simulink model "part2_MAIN_2019_for_ayon_because_he_cant_update_his_matlab"  (R2019a)
settings: Solver=FixedStepAuto  StartTime=0.0  StopTime=300  FixedStep=0.1  RelTol=1e-3
values from neighbouring files (symbols this model uses):
  Af = diag(ti)    [init.m]    (also in init_old.m)
  Aw = [zeros(3) eye(3) ... (first row only)    [get_observer_parameters.m]
  B = [thr1 thr2_x thr2_y thr3 thr4_x thr4_y thr5_x thr5_y]    [B_redistributed.m]    (also in check_alg.m = [1 2 3 4 5 6 7 8; get_observer_parameters.m = [zeros(6,3);zeros(3,3);zeros(3,3);inv(M)])
  change_position_time = 1200    [init.m]    (also in init_old.m)
  Cw = [zeros(3) eye(3)]    [get_observer_parameters.m]
  D = Damping    [init.m]    (also in init_old.m)
  Damping = diag([2.6486e5, 8.8164e5, 3.3774e8])    [init.m]    (also in init_old.m)
  direction_limit = pi/36    (= 0.0872664625997)    [init.m]    (also in init_old.m)
  direction_time_constant = 100    [init.m]    (also in init_old.m)
  dt = 0.1    [get_observer_parameters.m]
  E = [Ew, zeros(6,3) ... (first row only)    [get_observer_parameters.m]
  Gamma = diag(omega_is)    [init.m]    (also in init_old.m)
  gust_limit = 40    [init.m]    (also in init_old.m)
  H = [Cw, eye(3), zeros(3,3) zeros(3,3)]    [get_observer_parameters.m]    (also in quadprog.m = 2*diag([w.' w.' q.' q.' w_alpha.' w_alpha.']); quadprog_basic.m = 2*diag([w.' w.' q.' q.']); quadprog_false.m = 2*diag([w.' w.' q.' q.' w_alpha.' w_alpha.']))
  height = 3    [init.m]    (also in init_old.m)
  inv_M = inv(M)    [get_observer_parameters.m]
  inv_Tb = inv(Tb)    [get_observer_parameters.m]
  kappa = 0.003    [init.m]    (also in init_old.m)
  kappa2 = 0.0026    [init.m]    (also in init_old.m)
  Kd = [1660451.40544401; 3920391.80535684; 1605063439.04156]    [init.m]    (also in init_old.m)
  Ki = [137.081306245593; 3163.274947400198; 335358.448218978]    [init.m]    (also in init_old.m)
  Kp = [75459.3345349083; 277551.73586971; 120744473.878042]    [init.m]    (also in init_old.m)
  L = 1800    [init.m]    (also in init_old.m)
  M = Mass    [init.m]    (also in init_old.m)
  mean_wind_direction = pi    (= 3.14159265359)    [init.m]    (also in init_old.m)
  observer_type = 0    [init.m]    (also in init_old.m)
  Omega = diag([omega_n, omega_n, omega_n])    [get_observer_parameters.m]    (also in init.m = diag(2*omega_is.*zeta_is); init_old.m = diag(2*omega_is.*zeta_is))
  Q = diag([0.1,0.1,pi/180,1e6,1e6,1e9])*10e3    [get_observer_parameters.m]
  R = diag([1,0.1,0.1*pi/180])*10e-3    [get_observer_parameters.m]
  simulation = 7    [init.m]    (also in init_old.m = 1)
  slow_varying_limit = 1    [init.m]    (also in init_old.m)
  slow_varying_time_constant = 100    [init.m]    (also in init_old.m)
  TAU = dt*E    [get_observer_parameters.m]
  Tb = 0.1 * eye(3)    [get_observer_parameters.m]
  thruster_type = 0    [init.m]    (also in init_old.m)
  u10 = 12    [init.m]    (also in init_old.m)
  vessel =     [test.mat]
  wind = 1    [init.m]    (also in init_old.m)
undefined symbols (not defined in the file or in its folder): Hoerner, ModelParams, npf, Param, thrusters, WaveModel
libraries: simulink x49, dspsigops x39, marine_hydro x14, marine_gnc x7
(part 6 of 9)

== system part2_MAIN_2019_for_ayon_because_he_cant_update_his_matlab/Simulation 5/Observer/Passive Non-Linear ==
  note: eta_observer
  note: nu_observer
  note: Bias Estimator
  note: Wave Estimator: 1st order wave-induced motion
  y : Inport
  tau_est : Inport  Port=2
  Add : Sum
  Add1 : Sum  Inputs=++-
  Aw : Gain  Gain=WaveModel.A_w  Multiplication=Matrix(K*u)
  Cw : Gain  Gain=WaveModel.C_w  Multiplication=Matrix(K*u)
  Damping : Gain  Gain=Damping  Multiplication=Matrix(K*u)
  Integrator{,1..3} (4 alike) : Integrator
  K1 : Gain  Gain=npf.K_1  Multiplication=Matrix(K*u)
  K2 : Gain  Gain=npf.K_2  Multiplication=Matrix(K*u)
  K3 : Gain  Gain=npf.K_3  Multiplication=Matrix(K*u)
  K4 : Gain  Gain=npf.K_4  Multiplication=Matrix(K*u)
  M_inv : Gain  Gain=inv(ModelParams.Mass)  Multiplication=Matrix(K*u)
  Matrix Multiply : Product  Multiplication=Matrix(*)
  Matrix Multiply1 : Product  Multiplication=Matrix(*)
  Matrix Multiply2 : Product  Multiplication=Matrix(*)
  R_psi : MATLAB Function  TreatAsAtomicUnit=on
  R_psi_T : MATLAB Function  TreatAsAtomicUnit=on
  Subsystem : Subsystem
  Sum : Sum  Inputs=|++
  Sum1 : Sum  Inputs=|+-
  Sum2 : Sum  Inputs=|++
  Sum3 : Sum  Inputs=|++
  Sum4 : Sum  Inputs=|+-
  inv(Tb) : Gain  Gain=inv(Param.Tb)  Multiplication=Matrix(K*u)
  eta_hat : Outport
  nu_hat : Outport  Port=2
  wires:
  Matrix Multiply/1 -> Sum/1
  Matrix Multiply1/1 -> Add/2
  Matrix Multiply2/1 -> Add1/1  "R'b_hat"
  R_psi_T/1(y) -> Matrix Multiply/1, Matrix Multiply2/2
  Add1/1 -> M_inv/1
  Damping/1 -> Add1/3
  R_psi/1(y) -> Matrix Multiply1/1
  Sum/1 -> Add1/2  "R'k4y + tau"
  Add/1 -> Integrator3/1  "eta_hat_dot"
  inv(Tb)/1 -> Sum1/2
  y/1 -> Subsystem/1(y), Sum4/1  "y"
  Aw/1 -> Sum2/2
  K3/1 -> Sum1/1
  Cw/1 -> Sum3/1
  Integrator1/1 -> Cw/1, Aw/1  "zeta_hat"
  Sum1/1 -> Integrator2/1  "b_hat_dot"
  Integrator/1 -> nu_hat/1, Damping/1, Matrix Multiply1/2  "nu_hat"
  Sum4/1 -> K1/1, K2/1, K3/1, K4/1  "y_obs"
  Sum3/1 -> Sum4/2  "y_hat"
  Integrator3/1 -> eta_hat/1, Sum3/2  "eta_hat"
  Sum2/1 -> Integrator1/1
  K2/1 -> Add/1
  K4/1 -> Matrix Multiply/2
  M_inv/1 -> Integrator/1  "nu_hat_dot"
  Integrator2/1 -> inv(Tb)/1, Matrix Multiply2/1  "b_hat"
  tau_est/1 -> Sum/2
  K1/1 -> Sum2/1
  Subsystem/1(Out1) -> R_psi/1(u), R_psi_T/1(u)

== system part2_MAIN_2019_for_ayon_because_he_cant_update_his_matlab/Simulation 5/Observer/Subsystem ==
  In1 : Inport
  Demux : Demux  Outputs=6
  Mux : Mux  Inputs=3
  Terminator : Terminator
  Terminator1 : Terminator
  Terminator2 : Terminator
  Out1 : Outport
  wires:
  Mux/1 -> Out1/1
  Demux/6 -> Mux/3
  Demux/5 -> Terminator2/1
  Demux/2 -> Mux/2
  Demux/1 -> Mux/1
  Demux/3 -> Terminator/1
  In1/1 -> Demux/1
  Demux/4 -> Terminator1/1

== system part2_MAIN_2019_for_ayon_because_he_cant_update_his_matlab/Simulation 5/Reference Model/Simulation Selector ==
  Simulation 4 : Subsystem
  Out1 : Outport
  wires:
  Simulation 4/1(Out1) -> Out1/1

== system part2_MAIN_2019_for_ayon_because_he_cant_update_his_matlab/Simulation 5/Thrust Allocation/Unwrap ==
  alpha : Inport
  Demux : Demux  Outputs=5
  Mux : Mux  Inputs=5
  Unwrap : dspsigops/Unwrap  tol=pi  InputProcessing=Columns as channels (frame based)  running=off
  Unwrap1 : dspsigops/Unwrap  tol=pi  InputProcessing=Columns as channels (frame based)  running=off
  Unwrap2 : dspsigops/Unwrap  tol=pi  InputProcessing=Columns as channels (frame based)  running=off
  alpha [rad] : Outport
  wires:
  alpha/1 -> Demux/1
  Mux/1 -> alpha [rad]/1
  Demux/1 -> Mux/1
  Demux/4 -> Unwrap2/1
  Unwrap2/1 -> Mux/4
  Demux/5 -> Unwrap/1
  Unwrap/1 -> Mux/5
  Demux/3 -> Mux/3
  Demux/2 -> Unwrap1/1
  Unwrap1/1 -> Mux/2

== system part2_MAIN_2019_for_ayon_because_he_cant_update_his_matlab/Simulation 5/Thrust Allocation/Unwrap1 ==
  alpha : Inport
  Demux : Demux  Outputs=5
  Mux : Mux  Inputs=5
  Unwrap : dspsigops/Unwrap  tol=pi  InputProcessing=Columns as channels (frame based)  running=off
  Unwrap1 : dspsigops/Unwrap  tol=pi  InputProcessing=Columns as channels (frame based)  running=off
  Unwrap2 : dspsigops/Unwrap  tol=pi  InputProcessing=Columns as channels (frame based)  running=off
  alpha [rad] : Outport
  wires:
  Unwrap1/1 -> Mux/2
  Demux/2 -> Unwrap1/1
  Demux/3 -> Mux/3
  Unwrap/1 -> Mux/5
  Demux/5 -> Unwrap/1
  Unwrap2/1 -> Mux/4
  Demux/4 -> Unwrap2/1
  Demux/1 -> Mux/1
  Mux/1 -> alpha [rad]/1
  alpha/1 -> Demux/1

== system part2_MAIN_2019_for_ayon_because_he_cant_update_his_matlab/Simulation 5/Wind/V_w1 ==
  " " : Constant  Value=mean_wind_direction
  Band-Limited White Noise : simulink/Sources/Band-Limited White Noise  Cov=np_slow_varying  Ts=0.1  seed=[23341]
  Band-Limited White Noise1 : simulink/Sources/Band-Limited White Noise  Cov=np_direction  Ts=0.1  seed=[23341]
  Constant : Constant  Value=u10
  Constant1 : Constant  Value=kappa
  Constant2 : Constant  Value=height
  Constant3 : Constant  Value=u10
  Constant8 : Constant  Value=L
  Constant9 : Constant  Value=kappa2
  Gain : Gain  Gain=1/slow_varying_time_constant
  Gain1 : Gain  Gain=1/direction_time_constant
  Gust : MATLAB Function  TreatAsAtomicUnit=on
  Integrator : Integrator  LimitOutput=on  UpperSaturationLimit=slow_varying_limit  LowerSaturationLimit=-slow_varying_limit
  Integrator1 : Integrator  LimitOutput=on  UpperSaturationLimit=direction_limit  LowerSaturationLimit=-direction_limit
  Mean wind component : MATLAB Function  TreatAsAtomicUnit=on
  Saturation : Saturate  UpperLimit=gust_limit  LowerLimit=-10
  Scope{,1..3} (4 alike) : Scope
  Sum : Sum  Inputs=+|+|+
  Sum1 : Sum  Inputs=|+-
  Sum2 : Sum  Inputs=|+-
  Sum3 : Sum  Inputs=|++
  time : Clock
  wind : Outport
  direction : Outport  Port=2
  wires:
  Constant3/1 -> Mean wind component/1(u10)
  Constant1/1 -> Mean wind component/2(kappa)
  Constant2/1 -> Mean wind component/3(height)
  Mean wind component/1(mean_wind) -> Scope2/1, Sum/2
  Sum/1 -> wind/1
  Integrator/1 -> Scope1/1, Sum/1, Sum1/2
  Band-Limited White Noise/1 -> Sum1/1
  Integrator1/1 -> Sum2/2, Sum3/1
  Band-Limited White Noise1/1 -> Sum2/1
  " "/1 -> Sum3/2
  Sum3/1 -> Scope3/1, direction/1
  Gain1/1 -> Integrator1/1
  Sum2/1 -> Gain1/1
  Gain/1 -> Integrator/1
  Sum1/1 -> Gain/1
  Constant8/1 -> Gust/3(L)
  Gust/1(gust) -> Saturation/1
  Saturation/1 -> Sum/3, Scope/1
  Constant9/1 -> Gust/4(kappa2)
  Constant/1 -> Gust/2(u10)
  time/1 -> Gust/1(time)

== system part2_MAIN_2019_for_ayon_because_he_cant_update_his_matlab/Simulation 7/Current (North - East)/Subsystem ==
  Mux1 : Mux  Inputs=3
  Scope : Scope
  Step1 : Step  Time=0  After=0  SampleTime=0
  Step2 : Step  Time=0  After=-0.2  SampleTime=0
  Step3 : Step  Time=0  After=0  SampleTime=0
  Out1 : Outport
  wires:
  Mux1/1 -> Scope/1, Out1/1
  Step1/1 -> Mux1/1
  Step2/1 -> Mux1/2
  Step3/1 -> Mux1/3

== system part2_MAIN_2019_for_ayon_because_he_cant_update_his_matlab/Simulation 7/Current (North - East)/Subsystem1 ==
  Add : Sum  Inputs=+++
  Cos : Trigonometry  Operator=cos
  Gain : Gain  Gain=pi/180
  Matrix Multiply : Product
  Matrix Multiply1 : Product
  Mux : Mux  Inputs=3
  Ramp : simulink/Sources/Ramp  slope=0.45  start=2  InitialOutput=0
  Ramp1 : simulink/Sources/Ramp  slope=-0.45  start=202  InitialOutput=0
  Scope : Scope  NumInputPorts=3
  Sin : Trigonometry
  Step : Step  Time=2  After=0.5  SampleTime=0
  Step1 : Step  Time=2  Before=180  After=180  SampleTime=0
  Step2 : Step  Time=0  After=0  SampleTime=0
  Out1 : Outport
  wires:
  Step1/1 -> Add/1
  Ramp/1 -> Add/2
  Ramp1/1 -> Add/3
  Step/1 -> Matrix Multiply1/1, Matrix Multiply/1
  Sin/1 -> Matrix Multiply1/2, Scope/1
  Cos/1 -> Matrix Multiply/2, Scope/2
  Matrix Multiply/1 -> Mux/1
  Matrix Multiply1/1 -> Mux/2
  Step2/1 -> Mux/3
  Mux/1 -> Scope/3, Out1/1
  Add/1 -> Gain/1
  Gain/1 -> Sin/1, Cos/1

== system part2_MAIN_2019_for_ayon_because_he_cant_update_his_matlab/Simulation 7/Current (North - East)/Subsystem2 ==
  Mux : Mux  Inputs=3
  Step : Step  Time=0  After=0  SampleTime=0
  Out1 : Outport
  wires:
  Mux/1 -> Out1/1
  Step/1 -> Mux/3, Mux/2, Mux/1

== system part2_MAIN_2019_for_ayon_because_he_cant_update_his_matlab/Simulation 7/Observer/EKF ==
  note: selector
  y : Inport
  U : Inport  Port=2
  Constant : Constant  Value=M
  Constant1 : Constant  Value=D
  Constant10 : Constant  Value=Q
  Constant11 : Constant  Value=dt
  Constant12 : Constant  Value=inv_Tb
  Constant13 : Constant  Value=TAU
  Constant2 : Constant  Value=inv_M
  Constant3 : Constant  Value=Tb
  Constant4 : Constant  Value=Aw
  Constant5 : Constant  Value=Cw
  Constant6 : Constant  Value=B
  Constant7 : Constant  Value=H
  Constant8 : Constant  Value=E
  Constant9 : Constant  Value=R
  MATLAB Function : MATLAB Function  TreatAsAtomicUnit=on
  MATLAB Function1 : MATLAB Function  TreatAsAtomicUnit=on
  Memory : Memory  InitialCondition=zeros(15,1)
  Memory1 : Memory  InitialCondition=eye(15,15)
  Scope : Scope
  Scope2 : Scope
  Subsystem : Subsystem  Commented=on
  Subsystem1 : Subsystem  Commented=on
  Terminator : Terminator
  eta_hat : Outport
  nu_hat : Outport  Port=2
  wires:
  U/1 -> MATLAB Function/2(U)
  MATLAB Function1/1(eta_hat) -> eta_hat/1
  MATLAB Function/3(states_hat) -> MATLAB Function1/1(states_vector)
  MATLAB Function/4(error) -> Scope2/1
  y/1 -> MATLAB Function/1(y)
  MATLAB Function1/2(nu_hat) -> nu_hat/1
  MATLAB Function/2(states_update) -> Memory/1
  Constant/1 -> MATLAB Function/5(M)
  Constant1/1 -> MATLAB Function/6(D)
  Constant2/1 -> MATLAB Function/7(inv_M)
  Constant4/1 -> MATLAB Function/8(Aw)
  Constant3/1 -> MATLAB Function/9(Tb)
  Constant5/1 -> MATLAB Function/10(Cw)
  Constant8/1 -> MATLAB Function/11(E)
  Constant6/1 -> MATLAB Function/12(B)
  Constant7/1 -> MATLAB Function/13(H)
  Constant9/1 -> MATLAB Function/14(R)
  Constant10/1 -> MATLAB Function/15(Q)
  Constant11/1 -> MATLAB Function/16(dt)
  Constant12/1 -> MATLAB Function/17(inv_Tb)
  Constant13/1 -> MATLAB Function/18(TAU)
  Memory/1 -> MATLAB Function/4(states)
  MATLAB Function/1(P_update) -> Memory1/1, Scope/1
  Memory1/1 -> MATLAB Function/3(P)
  MATLAB Function/5(K) -> Terminator/1

== system part2_MAIN_2019_for_ayon_because_he_cant_update_his_matlab/Simulation 7/Observer/Passive Non-Linear ==
  note: eta_observer
  note: nu_observer
  note: Bias Estimator
  note: Wave Estimator: 1st order wave-induced motion
  y : Inport
  tau_est : Inport  Port=2
  Add : Sum
  Add1 : Sum  Inputs=++-
  Aw : Gain  Gain=WaveModel.A_w  Multiplication=Matrix(K*u)
  Cw : Gain  Gain=WaveModel.C_w  Multiplication=Matrix(K*u)
  Damping : Gain  Gain=Damping  Multiplication=Matrix(K*u)
  Integrator{,1..3} (4 alike) : Integrator
  K1 : Gain  Gain=npf.K_1  Multiplication=Matrix(K*u)
  K2 : Gain  Gain=npf.K_2  Multiplication=Matrix(K*u)
  K3 : Gain  Gain=npf.K_3  Multiplication=Matrix(K*u)
  K4 : Gain  Gain=npf.K_4  Multiplication=Matrix(K*u)
  M_inv : Gain  Gain=inv(ModelParams.Mass)  Multiplication=Matrix(K*u)
  Matrix Multiply : Product  Multiplication=Matrix(*)
  Matrix Multiply1 : Product  Multiplication=Matrix(*)
  Matrix Multiply2 : Product  Multiplication=Matrix(*)
  R_psi : MATLAB Function  TreatAsAtomicUnit=on
  R_psi_T : MATLAB Function  TreatAsAtomicUnit=on
  Subsystem : Subsystem
  Sum : Sum  Inputs=|++
  Sum1 : Sum  Inputs=|+-
  Sum2 : Sum  Inputs=|++
  Sum3 : Sum  Inputs=|++
  Sum4 : Sum  Inputs=|+-
  inv(Tb) : Gain  Gain=inv(Param.Tb)  Multiplication=Matrix(K*u)
  eta_hat : Outport
  nu_hat : Outport  Port=2
  wires:
  Matrix Multiply/1 -> Sum/1
  Matrix Multiply1/1 -> Add/2
  Matrix Multiply2/1 -> Add1/1  "R'b_hat"
  R_psi_T/1(y) -> Matrix Multiply/1, Matrix Multiply2/2
  Add1/1 -> M_inv/1
  Damping/1 -> Add1/3
  R_psi/1(y) -> Matrix Multiply1/1
  Sum/1 -> Add1/2  "R'k4y + tau"
  Add/1 -> Integrator3/1  "eta_hat_dot"
  inv(Tb)/1 -> Sum1/2
  y/1 -> Subsystem/1(y), Sum4/1  "y"
  Aw/1 -> Sum2/2
  K3/1 -> Sum1/1
  Cw/1 -> Sum3/1
  Integrator1/1 -> Cw/1, Aw/1  "zeta_hat"
  Sum1/1 -> Integrator2/1  "b_hat_dot"
  Integrator/1 -> nu_hat/1, Damping/1, Matrix Multiply1/2  "nu_hat"
  Sum4/1 -> K1/1, K2/1, K3/1, K4/1  "y_obs"
  Sum3/1 -> Sum4/2  "y_hat"
  Integrator3/1 -> eta_hat/1, Sum3/2  "eta_hat"
  Sum2/1 -> Integrator1/1
  K2/1 -> Add/1
  K4/1 -> Matrix Multiply/2
  M_inv/1 -> Integrator/1  "nu_hat_dot"
  Integrator2/1 -> inv(Tb)/1, Matrix Multiply2/1  "b_hat"
  tau_est/1 -> Sum/2
  K1/1 -> Sum2/1
  Subsystem/1(Out1) -> R_psi/1(u), R_psi_T/1(u)

== system part2_MAIN_2019_for_ayon_because_he_cant_update_his_matlab/Simulation 7/Observer/Subsystem ==
  In1 : Inport
  Demux : Demux  Outputs=6
  Mux : Mux  Inputs=3
  Terminator : Terminator
  Terminator1 : Terminator
  Terminator2 : Terminator
  Out1 : Outport
  wires:
  Mux/1 -> Out1/1
  Demux/6 -> Mux/3
  Demux/5 -> Terminator2/1
  Demux/2 -> Mux/2
  Demux/1 -> Mux/1
  Demux/3 -> Terminator/1
  In1/1 -> Demux/1
  Demux/4 -> Terminator1/1

== system part2_MAIN_2019_for_ayon_because_he_cant_update_his_matlab/Simulation 7/Reference Model/Simulation Selector ==
  Simulation 4 : Subsystem
  Out1 : Outport
  wires:
  Simulation 4/1(Out1) -> Out1/1

== system part2_MAIN_2019_for_ayon_because_he_cant_update_his_matlab/Simulation 7/Thrust Allocation/Unwrap ==
  alpha : Inport
  Demux : Demux  Outputs=5
  Mux : Mux  Inputs=5
  Unwrap : dspsigops/Unwrap  tol=pi  InputProcessing=Columns as channels (frame based)  running=off
  Unwrap1 : dspsigops/Unwrap  tol=pi  InputProcessing=Columns as channels (frame based)  running=off
  Unwrap2 : dspsigops/Unwrap  tol=pi  InputProcessing=Columns as channels (frame based)  running=off
  alpha [rad] : Outport
  wires:
  alpha/1 -> Demux/1
  Mux/1 -> alpha [rad]/1
  Demux/1 -> Mux/1
  Demux/4 -> Unwrap2/1
  Unwrap2/1 -> Mux/4
  Demux/5 -> Unwrap/1
  Unwrap/1 -> Mux/5
  Demux/3 -> Mux/3
  Demux/2 -> Unwrap1/1
  Unwrap1/1 -> Mux/2

== system part2_MAIN_2019_for_ayon_because_he_cant_update_his_matlab/Simulation 7/Thrust Allocation/Unwrap1 ==
  alpha : Inport
  Demux : Demux  Outputs=5
  Mux : Mux  Inputs=5
  Unwrap : dspsigops/Unwrap  tol=pi  InputProcessing=Columns as channels (frame based)  running=off
  Unwrap1 : dspsigops/Unwrap  tol=pi  InputProcessing=Columns as channels (frame based)  running=off
  Unwrap2 : dspsigops/Unwrap  tol=pi  InputProcessing=Columns as channels (frame based)  running=off
  alpha [rad] : Outport
  wires:
  Unwrap1/1 -> Mux/2
  Demux/2 -> Unwrap1/1
  Demux/3 -> Mux/3
  Unwrap/1 -> Mux/5
  Demux/5 -> Unwrap/1
  Unwrap2/1 -> Mux/4
  Demux/4 -> Unwrap2/1
  Demux/1 -> Mux/1
  Mux/1 -> alpha [rad]/1
  alpha/1 -> Demux/1

== system part2_MAIN_2019_for_ayon_because_he_cant_update_his_matlab/Simulation 7/Wind/V_w1 ==
  " " : Constant  Value=mean_wind_direction
  Band-Limited White Noise : simulink/Sources/Band-Limited White Noise  Cov=np_slow_varying  Ts=0.1  seed=[23341]
  Band-Limited White Noise1 : simulink/Sources/Band-Limited White Noise  Cov=np_direction  Ts=0.1  seed=[23341]
  Constant : Constant  Value=u10
  Constant1 : Constant  Value=kappa
  Constant2 : Constant  Value=height
  Constant3 : Constant  Value=u10
  Constant8 : Constant  Value=L
  Constant9 : Constant  Value=kappa2
  Gain : Gain  Gain=1/slow_varying_time_constant
  Gain1 : Gain  Gain=1/direction_time_constant
  Gust : MATLAB Function  TreatAsAtomicUnit=on
  Integrator : Integrator  LimitOutput=on  UpperSaturationLimit=slow_varying_limit  LowerSaturationLimit=-slow_varying_limit
  Integrator1 : Integrator  LimitOutput=on  UpperSaturationLimit=direction_limit  LowerSaturationLimit=-direction_limit
  Mean wind component : MATLAB Function  TreatAsAtomicUnit=on
  Saturation : Saturate  UpperLimit=gust_limit  LowerLimit=-10
  Scope{,1..3} (4 alike) : Scope
  Sum : Sum  Inputs=+|+|+
  Sum1 : Sum  Inputs=|+-
  Sum2 : Sum  Inputs=|+-
  Sum3 : Sum  Inputs=|++
  time : Clock
  wind : Outport
  direction : Outport  Port=2
  wires:
  Constant3/1 -> Mean wind component/1(u10)
  Constant1/1 -> Mean wind component/2(kappa)
  Constant2/1 -> Mean wind component/3(height)
  Mean wind component/1(mean_wind) -> Scope2/1, Sum/2
  Sum/1 -> wind/1
  Integrator/1 -> Scope1/1, Sum/1, Sum1/2
  Band-Limited White Noise/1 -> Sum1/1
  Integrator1/1 -> Sum2/2, Sum3/1
  Band-Limited White Noise1/1 -> Sum2/1
  " "/1 -> Sum3/2
  Sum3/1 -> Scope3/1, direction/1
  Gain1/1 -> Integrator1/1
  Sum2/1 -> Gain1/1
  Gain/1 -> Integrator/1
  Sum1/1 -> Gain/1
  Constant8/1 -> Gust/3(L)
  Gust/1(gust) -> Saturation/1
  Saturation/1 -> Sum/3, Scope/1
  Constant9/1 -> Gust/4(kappa2)
  Constant/1 -> Gust/2(u10)
  time/1 -> Gust/1(time)

== system part2_MAIN_2019_for_ayon_because_he_cant_update_his_matlab/ Original/Observer/EKF/Subsystem ==
  note: simulation time
  note: P_selector
  In1 : Inport
  In2 : Inport  Port=2
  Constant1 : Constant  Value=eye(15)
  Constant2 : Constant  Value=zeros(15,1)
  Step : Step  Time=0.01  SampleTime=0.1
  Switch : Switch  Threshold=1
  Switch1 : Switch  Threshold=1
  Out1 : Outport
  Out2 : Outport  Port=2
  wires:
  Switch1/1 -> Out2/1
  In1/1 -> Switch/1
  In2/1 -> Switch1/1
  Switch/1 -> Out1/1
  Constant1/1 -> Switch/3
  Step/1 -> Switch1/2, Switch/2
  Constant2/1 -> Switch1/3

== system part2_MAIN_2019_for_ayon_because_he_cant_update_his_matlab/ Original/Observer/EKF/Subsystem1 ==
  note: P
  note: states
  note: simulation time
  States : Inport
  P : Inport  Port=2
  MATLAB Function : MATLAB Function  TreatAsAtomicUnit=on
  Step1 : Step  Time=0.01  After=10  SampleTime=0.1
  states1 : Outport
  P1 : Outport  Port=2
  wires:
  Step1/1 -> MATLAB Function/1(u)
  P/1 -> MATLAB Function/2(P)
  States/1 -> MATLAB Function/3(states)
  MATLAB Function/1(P1) -> P1/1
  MATLAB Function/2(states1) -> states1/1

== system part2_MAIN_2019_for_ayon_because_he_cant_update_his_matlab/ Original/Observer/Passive Non-Linear/Subsystem ==
  y : Inport
  Demux : Demux  Outputs=3
  Terminator : Terminator
  Terminator1 : Terminator
  Out1 : Outport
  wires:
  y/1 -> Demux/1
  Demux/3 -> Out1/1
  Demux/1 -> Terminator/1
  Demux/2 -> Terminator1/1

== system part2_MAIN_2019_for_ayon_because_he_cant_update_his_matlab/ Original/Reference Model/Simulation Selector/Subsystem ==
  note: yaw
  note: sway
  note: surge
  Mux : Mux  Inputs=3
  Scope : Scope
  Step : Step  After=10  SampleTime=0
  Step1 : Step  After=10  SampleTime=0
  Step2 : Step  After=3*pi/2  SampleTime=0
  Set-point : Outport
  wires:
  Step/1 -> Mux/1
  Step1/1 -> Mux/2
  Step2/1 -> Mux/3
  Mux/1 -> Scope/1, Set-point/1

== system part2_MAIN_2019_for_ayon_because_he_cant_update_his_matlab/ Original/Reference Model/Simulation Selector/Subsystem1 ==
  note: yaw
  note: sway
  note: surge
  Add : Sum
  Add1 : Sum
  Add2 : Sum
  Mux : Mux  Inputs=3
  Scope : Scope
  Step : Step  Time=10  After=50  SampleTime=0
  Step1 : Step  Time=change_position_time  After=-50  SampleTime=0
  Step2 : Step  Time=change_position_time*2  After=pi/4  SampleTime=0
  Step3 : Step  Time=change_position_time*3  After=-50  SampleTime=0
  Step4 : Step  Time=change_position_time*4  After=50  SampleTime=0
  Step5 : Step  Time=change_position_time*4  After=-pi/4  SampleTime=0
  Out1 : Outport
  wires:
  Mux/1 -> Scope/1, Out1/1
  Step/1 -> Add/1
  Step3/1 -> Add/2
  Step1/1 -> Add1/1
  Step4/1 -> Add1/2
  Step2/1 -> Add2/1
  Step5/1 -> Add2/2
  Add/1 -> Mux/1
  Add1/1 -> Mux/2
  Add2/1 -> Mux/3

== system part2_MAIN_2019_for_ayon_because_he_cant_update_his_matlab/ Original/Reference Model/Simulation Selector/Subsystem2 ==
  Mux : Mux  Inputs=3
  Step : Step  After=0  SampleTime=0
  Step1 : Step  After=0  SampleTime=0
  Step2 : Step  After=0  SampleTime=0
  Out1 : Outport
  wires:
  Step/1 -> Mux/1
  Step1/1 -> Mux/2
  Step2/1 -> Mux/3
  Mux/1 -> Out1/1

== system part2_MAIN_2019_for_ayon_because_he_cant_update_his_matlab/Simulation 1/Observer/EKF/Subsystem ==
  note: simulation time
  note: P_selector
  In1 : Inport
  In2 : Inport  Port=2
  Constant1 : Constant  Value=eye(15)
  Constant2 : Constant  Value=zeros(15,1)
  Step : Step  Time=0.01  SampleTime=0.1
  Switch : Switch  Threshold=1
  Switch1 : Switch  Threshold=1
  Out1 : Outport
  Out2 : Outport  Port=2
  wires:
  Switch1/1 -> Out2/1
  In1/1 -> Switch/1
  In2/1 -> Switch1/1
  Switch/1 -> Out1/1
  Constant1/1 -> Switch/3
  Step/1 -> Switch1/2, Switch/2
  Constant2/1 -> Switch1/3

== system part2_MAIN_2019_for_ayon_because_he_cant_update_his_matlab/Simulation 1/Observer/EKF/Subsystem1 ==
  note: P
  note: states
  note: simulation time
  States : Inport
  P : Inport  Port=2
  MATLAB Function : MATLAB Function  TreatAsAtomicUnit=on
  Step1 : Step  Time=0.01  After=10  SampleTime=0.1
  states1 : Outport
  P1 : Outport  Port=2
  wires:
  Step1/1 -> MATLAB Function/1(u)
  P/1 -> MATLAB Function/2(P)
  States/1 -> MATLAB Function/3(states)
  MATLAB Function/1(P1) -> P1/1
  MATLAB Function/2(states1) -> states1/1

== system part2_MAIN_2019_for_ayon_because_he_cant_update_his_matlab/Simulation 1/Observer/Passive Non-Linear/Subsystem ==
  y : Inport
  Demux : Demux  Outputs=3
  Terminator : Terminator
  Terminator1 : Terminator
  Out1 : Outport
  wires:
  y/1 -> Demux/1
  Demux/3 -> Out1/1
  Demux/1 -> Terminator/1
  Demux/2 -> Terminator1/1

== system part2_MAIN_2019_for_ayon_because_he_cant_update_his_matlab/Simulation 1/Reference Model/Simulation Selector/Simulation 4 ==
  note: yaw
  note: sway
  note: surge
  Add : Sum
  Add1 : Sum
  Add2 : Sum
  Mux : Mux  Inputs=3
  Scope : Scope
  Step : Step  Time=0  After=50  SampleTime=0
  Step1 : Step  Time=change_position_time  After=-50  SampleTime=0
  Step2 : Step  Time=change_position_time*2  After=pi/4  SampleTime=0
  Step3 : Step  Time=change_position_time*3  After=-50  SampleTime=0
  Step4 : Step  Time=change_position_time*4  After=50  SampleTime=0
  Step5 : Step  Time=change_position_time*4  After=-pi/4  SampleTime=0
  Out1 : Outport
  wires:
  Mux/1 -> Scope/1, Out1/1
  Step/1 -> Add/1
  Step3/1 -> Add/2
  Step1/1 -> Add1/1
  Step4/1 -> Add1/2
  Step2/1 -> Add2/1
  Step5/1 -> Add2/2
  Add/1 -> Mux/1
  Add1/1 -> Mux/2
  Add2/1 -> Mux/3

== system part2_MAIN_2019_for_ayon_because_he_cant_update_his_matlab/Simulation 2/Observer/EKF/Subsystem ==
  note: simulation time
  note: P_selector
  In1 : Inport
  In2 : Inport  Port=2
  Constant1 : Constant  Value=eye(15)
  Constant2 : Constant  Value=zeros(15,1)
  Step : Step  Time=0.01  SampleTime=0.1
  Switch : Switch  Threshold=1
  Switch1 : Switch  Threshold=1
  Out1 : Outport
  Out2 : Outport  Port=2
  wires:
  Switch1/1 -> Out2/1
  In1/1 -> Switch/1
  In2/1 -> Switch1/1
  Switch/1 -> Out1/1
  Constant1/1 -> Switch/3
  Step/1 -> Switch1/2, Switch/2
  Constant2/1 -> Switch1/3

== system part2_MAIN_2019_for_ayon_because_he_cant_update_his_matlab/Simulation 2/Observer/EKF/Subsystem1 ==
  note: P
  note: states
  note: simulation time
  States : Inport
  P : Inport  Port=2
  MATLAB Function : MATLAB Function  TreatAsAtomicUnit=on
  Step1 : Step  Time=0.01  After=10  SampleTime=0.1
  states1 : Outport
  P1 : Outport  Port=2
  wires:
  Step1/1 -> MATLAB Function/1(u)
  P/1 -> MATLAB Function/2(P)
  States/1 -> MATLAB Function/3(states)
  MATLAB Function/1(P1) -> P1/1
  MATLAB Function/2(states1) -> states1/1

== system part2_MAIN_2019_for_ayon_because_he_cant_update_his_matlab/Simulation 2/Observer/Passive Non-Linear/Subsystem ==
  y : Inport
  Demux : Demux  Outputs=3
  Terminator : Terminator
  Terminator1 : Terminator
  Out1 : Outport
  wires:
  y/1 -> Demux/1
  Demux/3 -> Out1/1
  Demux/1 -> Terminator/1
  Demux/2 -> Terminator1/1

== system part2_MAIN_2019_for_ayon_because_he_cant_update_his_matlab/Simulation 2/Reference Model/Simulation Selector/Simulation 4 ==
  note: yaw
  note: sway
  note: surge
  Add : Sum
  Add1 : Sum
  Add2 : Sum
  Mux : Mux  Inputs=3
  Scope : Scope
  Step : Step  Time=0  After=50  SampleTime=0
  Step1 : Step  Time=change_position_time  After=-50  SampleTime=0
  Step2 : Step  Time=change_position_time*2  After=pi/4  SampleTime=0
  Step3 : Step  Time=change_position_time*3  After=-50  SampleTime=0
  Step4 : Step  Time=change_position_time*4  After=50  SampleTime=0
  Step5 : Step  Time=change_position_time*4  After=-pi/4  SampleTime=0
  Out1 : Outport
  wires:
  Mux/1 -> Scope/1, Out1/1
  Step/1 -> Add/1
  Step3/1 -> Add/2
  Step1/1 -> Add1/1
  Step4/1 -> Add1/2
  Step2/1 -> Add2/1
  Step5/1 -> Add2/2
  Add/1 -> Mux/1
  Add1/1 -> Mux/2
  Add2/1 -> Mux/3

== system part2_MAIN_2019_for_ayon_because_he_cant_update_his_matlab/Simulation 3/Observer/EKF/Subsystem ==
  note: simulation time
  note: P_selector
  In1 : Inport
  In2 : Inport  Port=2
  Constant1 : Constant  Value=eye(15)
  Constant2 : Constant  Value=zeros(15,1)
  Step : Step  Time=0.01  SampleTime=0.1
  Switch : Switch  Threshold=1
  Switch1 : Switch  Threshold=1
  Out1 : Outport
  Out2 : Outport  Port=2
  wires:
  Switch1/1 -> Out2/1
  In1/1 -> Switch/1
  In2/1 -> Switch1/1
  Switch/1 -> Out1/1
  Constant1/1 -> Switch/3
  Step/1 -> Switch1/2, Switch/2
  Constant2/1 -> Switch1/3

== system part2_MAIN_2019_for_ayon_because_he_cant_update_his_matlab/Simulation 3/Observer/EKF/Subsystem1 ==
  note: P
  note: states
  note: simulation time
  States : Inport
  P : Inport  Port=2
  MATLAB Function : MATLAB Function  TreatAsAtomicUnit=on
  Step1 : Step  Time=0.01  After=10  SampleTime=0.1
  states1 : Outport
  P1 : Outport  Port=2
  wires:
  Step1/1 -> MATLAB Function/1(u)
  P/1 -> MATLAB Function/2(P)
  States/1 -> MATLAB Function/3(states)
  MATLAB Function/1(P1) -> P1/1
  MATLAB Function/2(states1) -> states1/1

== system part2_MAIN_2019_for_ayon_because_he_cant_update_his_matlab/Simulation 3/Observer/Passive Non-Linear/Subsystem ==
  y : Inport
  Demux : Demux  Outputs=3
  Terminator : Terminator
  Terminator1 : Terminator
  Out1 : Outport
  wires:
  y/1 -> Demux/1
  Demux/3 -> Out1/1
  Demux/1 -> Terminator/1
  Demux/2 -> Terminator1/1

== system part2_MAIN_2019_for_ayon_because_he_cant_update_his_matlab/Simulation 3/Reference Model/Simulation Selector/Simulation 4 ==
  note: yaw
  note: sway
  note: surge
  Add : Sum
  Add1 : Sum
  Add2 : Sum
  Mux : Mux  Inputs=3
  Scope : Scope
  Step : Step  Time=0  After=50  SampleTime=0
  Step1 : Step  Time=change_position_time  After=-50  SampleTime=0
  Step2 : Step  Time=change_position_time*2  After=pi/4  SampleTime=0
  Step3 : Step  Time=change_position_time*3  After=-50  SampleTime=0
  Step4 : Step  Time=change_position_time*4  After=50  SampleTime=0
  Step5 : Step  Time=change_position_time*4  After=-pi/4  SampleTime=0
  Out1 : Outport
  wires:
  Mux/1 -> Scope/1, Out1/1
  Step/1 -> Add/1
  Step3/1 -> Add/2
  Step1/1 -> Add1/1
  Step4/1 -> Add1/2
  Step2/1 -> Add2/1
  Step5/1 -> Add2/2
  Add/1 -> Mux/1
  Add1/1 -> Mux/2
  Add2/1 -> Mux/3

== system part2_MAIN_2019_for_ayon_because_he_cant_update_his_matlab/Simulation 4/Observer/EKF/Subsystem ==
  note: simulation time
  note: P_selector
  In1 : Inport
  In2 : Inport  Port=2
  Constant1 : Constant  Value=eye(15)
  Constant2 : Constant  Value=zeros(15,1)
  Step : Step  Time=0.01  SampleTime=0.1
  Switch : Switch  Threshold=1
  Switch1 : Switch  Threshold=1
  Out1 : Outport
  Out2 : Outport  Port=2
  wires:
  Switch1/1 -> Out2/1
  In1/1 -> Switch/1
  In2/1 -> Switch1/1
  Switch/1 -> Out1/1
  Constant1/1 -> Switch/3
  Step/1 -> Switch1/2, Switch/2
  Constant2/1 -> Switch1/3

== system part2_MAIN_2019_for_ayon_because_he_cant_update_his_matlab/Simulation 4/Observer/EKF/Subsystem1 ==
  note: P
  note: states
  note: simulation time
  States : Inport
  P : Inport  Port=2
  MATLAB Function : MATLAB Function  TreatAsAtomicUnit=on
  Step1 : Step  Time=0.01  After=10  SampleTime=0.1
  states1 : Outport
  P1 : Outport  Port=2
  wires:
  Step1/1 -> MATLAB Function/1(u)
  P/1 -> MATLAB Function/2(P)
  States/1 -> MATLAB Function/3(states)
  MATLAB Function/1(P1) -> P1/1
  MATLAB Function/2(states1) -> states1/1

== system part2_MAIN_2019_for_ayon_because_he_cant_update_his_matlab/Simulation 4/Observer/Passive Non-Linear/Subsystem ==
  y : Inport
  Demux : Demux  Outputs=3
  Terminator : Terminator
  Terminator1 : Terminator
  Out1 : Outport
  wires:
  y/1 -> Demux/1
  Demux/3 -> Out1/1
  Demux/1 -> Terminator/1
  Demux/2 -> Terminator1/1

== system part2_MAIN_2019_for_ayon_because_he_cant_update_his_matlab/Simulation 4/Reference Model/Simulation Selector/Simulation 4 ==
  note: yaw
  note: sway
  note: surge
  Add : Sum
  Add1 : Sum
  Add2 : Sum
  Mux : Mux  Inputs=3
  Scope : Scope
  Step : Step  Time=0  After=50  SampleTime=0
  Step1 : Step  Time=change_position_time  After=-50  SampleTime=0
  Step2 : Step  Time=change_position_time*2  After=pi/4  SampleTime=0
  Step3 : Step  Time=change_position_time*3  After=-50  SampleTime=0
  Step4 : Step  Time=change_position_time*4  After=50  SampleTime=0
  Step5 : Step  Time=change_position_time*4  After=-pi/4  SampleTime=0
  Out1 : Outport
  wires:
  Mux/1 -> Scope/1, Out1/1
  Step/1 -> Add/1
  Step3/1 -> Add/2
  Step1/1 -> Add1/1
  Step4/1 -> Add1/2
  Step2/1 -> Add2/1
  Step5/1 -> Add2/2
  Add/1 -> Mux/1
  Add1/1 -> Mux/2
  Add2/1 -> Mux/3

== system part2_MAIN_2019_for_ayon_because_he_cant_update_his_matlab/Simulation 5/Observer/EKF/Subsystem ==
  note: simulation time
  note: P_selector
  In1 : Inport
  In2 : Inport  Port=2
  Constant1 : Constant  Value=eye(15)
  Constant2 : Constant  Value=zeros(15,1)
  Step : Step  Time=0.01  SampleTime=0.1
  Switch : Switch  Threshold=1
  Switch1 : Switch  Threshold=1
  Out1 : Outport
  Out2 : Outport  Port=2
  wires:
  Switch1/1 -> Out2/1
  In1/1 -> Switch/1
  In2/1 -> Switch1/1
  Switch/1 -> Out1/1
  Constant1/1 -> Switch/3
  Step/1 -> Switch1/2, Switch/2
  Constant2/1 -> Switch1/3

== system part2_MAIN_2019_for_ayon_because_he_cant_update_his_matlab/Simulation 5/Observer/EKF/Subsystem1 ==
  note: P
  note: states
  note: simulation time
  States : Inport
  P : Inport  Port=2
  MATLAB Function : MATLAB Function  TreatAsAtomicUnit=on
  Step1 : Step  Time=0.01  After=10  SampleTime=0.1
  states1 : Outport
  P1 : Outport  Port=2
  wires:
  Step1/1 -> MATLAB Function/1(u)
  P/1 -> MATLAB Function/2(P)
  States/1 -> MATLAB Function/3(states)
  MATLAB Function/1(P1) -> P1/1
  MATLAB Function/2(states1) -> states1/1

== system part2_MAIN_2019_for_ayon_because_he_cant_update_his_matlab/Simulation 5/Observer/Passive Non-Linear/Subsystem ==
  y : Inport
  Demux : Demux  Outputs=3
  Terminator : Terminator
  Terminator1 : Terminator
  Out1 : Outport
  wires:
  y/1 -> Demux/1
  Demux/3 -> Out1/1
  Demux/1 -> Terminator/1
  Demux/2 -> Terminator1/1

== system part2_MAIN_2019_for_ayon_because_he_cant_update_his_matlab/Simulation 5/Reference Model/Simulation Selector/Simulation 4 ==
  note: yaw
  note: sway
  note: surge
  Add : Sum
  Add1 : Sum
  Add2 : Sum
  Mux : Mux  Inputs=3
  Scope : Scope
  Step : Step  Time=0  After=50  SampleTime=0
  Step1 : Step  Time=change_position_time  After=-50  SampleTime=0
  Step2 : Step  Time=change_position_time*2  After=pi/4  SampleTime=0
  Step3 : Step  Time=change_position_time*3  After=-50  SampleTime=0
  Step4 : Step  Time=change_position_time*4  After=50  SampleTime=0
  Step5 : Step  Time=change_position_time*4  After=-pi/4  SampleTime=0
  Out1 : Outport
  wires:
  Mux/1 -> Scope/1, Out1/1
  Step/1 -> Add/1
  Step3/1 -> Add/2
  Step1/1 -> Add1/1
  Step4/1 -> Add1/2
  Step2/1 -> Add2/1
  Step5/1 -> Add2/2
  Add/1 -> Mux/1
  Add1/1 -> Mux/2
  Add2/1 -> Mux/3

== system part2_MAIN_2019_for_ayon_because_he_cant_update_his_matlab/Simulation 7/Observer/EKF/Subsystem ==
  note: simulation time
  note: P_selector
  In1 : Inport
  In2 : Inport  Port=2
  Constant1 : Constant  Value=eye(15)
  Constant2 : Constant  Value=zeros(15,1)
  Step : Step  Time=0.01  SampleTime=0.1
  Switch : Switch  Threshold=1
  Switch1 : Switch  Threshold=1
  Out1 : Outport
  Out2 : Outport  Port=2
  wires:
  Switch1/1 -> Out2/1
  In1/1 -> Switch/1
  In2/1 -> Switch1/1
  Switch/1 -> Out1/1
  Constant1/1 -> Switch/3
  Step/1 -> Switch1/2, Switch/2
  Constant2/1 -> Switch1/3

== system part2_MAIN_2019_for_ayon_because_he_cant_update_his_matlab/Simulation 7/Observer/EKF/Subsystem1 ==
  note: P
  note: states
  note: simulation time
  States : Inport
  P : Inport  Port=2
  MATLAB Function : MATLAB Function  TreatAsAtomicUnit=on
  Step1 : Step  Time=0.01  After=10  SampleTime=0.1
  states1 : Outport
  P1 : Outport  Port=2
  wires:
  Step1/1 -> MATLAB Function/1(u)
  P/1 -> MATLAB Function/2(P)
  States/1 -> MATLAB Function/3(states)
  MATLAB Function/1(P1) -> P1/1
  MATLAB Function/2(states1) -> states1/1

== system part2_MAIN_2019_for_ayon_because_he_cant_update_his_matlab/Simulation 7/Observer/Passive Non-Linear/Subsystem ==
  y : Inport
  Demux : Demux  Outputs=3
  Terminator : Terminator
  Terminator1 : Terminator
  Out1 : Outport
  wires:
  y/1 -> Demux/1
  Demux/3 -> Out1/1
  Demux/1 -> Terminator/1
  Demux/2 -> Terminator1/1

== system part2_MAIN_2019_for_ayon_because_he_cant_update_his_matlab/Simulation 7/Reference Model/Simulation Selector/Simulation 4 ==
  note: yaw
  note: sway
  Mux : Mux  Inputs=3
  Scope : Scope
  Step : Step  Time=0  After=0  SampleTime=0
  Step4 : Step  Time=0  After=0  SampleTime=0
  Step5 : Step  Time=0  After=0  SampleTime=0
  Out1 : Outport
  wires:
  Step/1 -> Mux/1
  Mux/1 -> Scope/1, Out1/1
  Step4/1 -> Mux/2
  Step5/1 -> Mux/3

== matlab function part2_MAIN_2019_for_ayon_because_he_cant_update_his_matlab/ Original/Current (North - East)/MATLAB Function ==
  data: u input; y output
function y = fcn(u)
rot = [cos(u) -sin(u) 0;
    sin(u) cos(u) 0;
    0 0 1];

y = rot';

== matlab function part2_MAIN_2019_for_ayon_because_he_cant_update_his_matlab/ Original/DP Controller/MATLAB Function ==
  data: u input; y output
function y = fcn(u)

rot = [cos(u) -sin(u) 0;
    sin(u) cos(u) 0;
    0 0 1];

y = rot';

== matlab function part2_MAIN_2019_for_ayon_because_he_cant_update_his_matlab/ Original/DP Controller/MATLAB Function1 ==
  data: u input; y output
function y = fcn(u)

rot = [cos(u) -sin(u) 0;
    sin(u) cos(u) 0;
    0 0 1];

y = rot';

== matlab function part2_MAIN_2019_for_ayon_because_he_cant_update_his_matlab/ Original/Thruster Dynamics/MATLAB Function ==
  data: alpha_actual input; thrust_actual input; actual_tau output; PosX input; PosY input
function actual_tau   = fcn(alpha_actual,thrust_actual,PosX,PosY)

    Alpha_surge =[cos(alpha_actual(1)) cos(alpha_actual(2)) cos(alpha_actual(3)) cos(alpha_actual(4)) cos(alpha_actual(5))];  
    Alpha_sway = [sin(alpha_actual(1)) sin(alpha_actual(2)) sin(alpha_actual(3)) sin(alpha_actual(4)) sin(alpha_actual(5))];
    Alpha_yaw = [sin(alpha_actual(1))*PosX(1)-cos(alpha_actual(1))*PosY(1) sin(alpha_actual(2))*PosX(2)-cos(alpha_actual(2))*PosY(2) ...
                 sin(alpha_actual(3))*PosX(3)-cos(alpha_actual(3))*PosY(3) sin(alpha_actual(4))*PosX(4)-cos(alpha_actual(4))*PosY(4) ...
                 sin(alpha_actual(5))*PosX(5)-cos(alpha_actual(5))*PosY(5)];

    actual_tau = [Alpha_surge; Alpha_sway; Alpha_yaw]*thrust_actual;
end

== matlab function part2_MAIN_2019_for_ayon_because_he_cant_update_his_matlab/ Original/Observer/Passive Non-Linear/R_psi_T ==
  data: u input; y output
function y = fcn(u)

rot = [cos(u) -sin(u) 0;
    sin(u) cos(u) 0;
    0 0 1];

y = rot';

== matlab function part2_MAIN_2019_for_ayon_because_he_cant_update_his_matlab/ Original/Observer/Passive Non-Linear/R_psi ==
  data: u input; y output
function y = fcn(u)

rot = [cos(u) -sin(u) 0;
    sin(u) cos(u) 0;
    0 0 1];

y = rot;

== matlab function part2_MAIN_2019_for_ayon_because_he_cant_update_his_matlab/ Original/Thrust Allocation/MATLAB Function ==
  data: tau_d input; Td output; alpha output
function [Td, alpha] = p_inv_B(tau_d)
%% Build the B matrix
% Thruster 1
x1 = 39.3;
y1 = 0;
% Thruster 2
x2 = 35.6;
y2 = 0;
% Thruster 3
x3 = 31.3;
y3 = 0;
% Thruster 4
x4 = -28.5;
y4 = 5;
% Thruster 5
x5 = -28.5;
y5 = -5;

% Redistributed force for each thruster
thr1 = [0 1 x1].';
thr2_x = [1 0 y2].';
thr2_y = [0 1 x2].';
thr3 = [0 1 x3].';
thr4_x = [1 0 y4].';
thr4_y = [0 1 x4].';
thr5_x = [1 0 y5].';
thr5_y = [0 1 x5].';

% B redistributed
B = [thr1 thr2_x thr2_y thr3 thr4_x thr4_y thr5_x thr5_y];

%% Result
tau = [tau_d(1); tau_d(2); tau_d(6)];

Td_r = pinv(B) * tau;

% Thruster control
Td = [Td_r(1); 
      sqrt(Td_r(2)^2 + Td_r(3)^2); 
      Td_r(4); 
      sqrt(Td_r(5)^2 + Td_r(6)^2);
      sqrt(Td_r(7)^2 + Td_r(8)^2)];

% Thruster angle
% if Td_r(2) == 0
%     alpha2 = pi/2;
% else
%     alpha2 = atan(Td_r(3)/Td_r(2));
% end
% if Td_r(5) == 0
%     alpha4 = pi/2;
% else
%     alpha4 = atan(Td_r(6)/Td_r(5));
% end
% if Td_r(7) == 0
%     alpha5 = pi/2;
% else
%     alpha5 = atan(Td_r(8)/Td_r(7));
% end

alpha2 = atan2(Td_r(3),Td_r(2));
alpha4 = atan2(Td_r(6),Td_r(5));
alpha5 = atan2(Td_r(8),Td_r(7));

%atan2(num,den)

% alpha2 = atan(Td_r(3)/Td_r(2));
% alpha4 = atan(Td_r(6)/Td_r(5));
% alpha5 = atan(Td_r(8)/Td_r(7));

alpha = [pi/2; alpha2; pi/2; alpha4; alpha5];
end

== matlab function part2_MAIN_2019_for_ayon_because_he_cant_update_his_matlab/ Original/Observer/EKF/MATLAB Function ==
  data: y input; U input; P input; P_update output; states input; states_update output; states_hat output; error output; M input; D input; inv_M input; Aw input; Tb input; Cw input; E input; B input; H input; R input; Q input; dt input; inv_Tb input; TAU input; K output
function [P_update, states_update,states_hat,error, K]= fcn(y, U, P, states,M,D,inv_M, Aw,Tb,Cw,E,B,H,R,Q,dt, inv_Tb, TAU)
%%%P - 15x15
%states [zeta,eta, b, nu] --15x1
%zeta - 6x1, 
%eta - 3x1, 
%b - 3x1, 
%nu - 3x1
%u - 3x1 force input 

%Aw, Tb, B, E, H
%%%states
zeta = states(1:6,:);
eta = states(7:9,:);
b = states(10:12,:);
nu = states(13:15,:);

u = nu(1,1);
v = nu(2,1);
b_x = b(1,1);
b_y = b(2,1);


%% calculating FXU

Rot_R = [cos(eta(3,1)) -sin(eta(3,1)) 0;
    sin(eta(3,1)) cos(eta(3,1)) 0;
    0 0 1];

Fx = [
Aw*zeta;
Rot_R*nu;
-inv_Tb*b;
% zeros(3,1);
-inv_M*D*nu + inv_M*Rot_R'*b
];

F = zeros(15,1);
F = (B*U);
F = Fx +F;


%%

%predictor
%%phi = PHI(states,ws_var.dt, ws_var);
%calculating phi
A = zeros(15,15);
psi = eta(3,1);

% A(7,9) = -v*cos(psi)-u*sin(psi);
% A(7,13) = cos(psi);
% A(1,15) = 0;
% A(1,4) = 1;
% A(2,5) = 1;
% A(3,6) = 1;
% A(4,1) = -0.0987;
% A(4,4) = -0.0628;
% A(5,2) = -0.0987;
% A(5,5) = -0.0628;
% A(6,3) = -0.0987;
% A(6,6) = -0.0628;
% A(7,14) = -sin(psi);
% 
% A(8,9) = u*cos(psi)-v*sin(psi);
% A(8,13) = sin(psi);
% A(8,14) = cos(psi);
% A(9,15) = 1;
% A(10:12, 10:12) = -10*eye(3);
% A(13,9) = -1.43e-7*(b_y*cos(psi)+b_x*sin(psi));
% A(13,10) = 1.43e-7*cos(psi);
% A(13,11) = -1.43e-7*sin(psi);
% 
% A(14,9) = 1.17e-7*(b_x*cos(psi) - b_y*sin(psi));
% A(14,10) = 1.17e-7*sin(psi);
% A(14,11) = -1.46e-11;
% A(14,12) = 2.63e-10;
% 
% A(15,9) = 1.46e-11*(b_y*sin(psi) - b_x*cos(psi));
% A(15,10) = -1.46e-11*sin(psi);
% A(15,11) = -1.46e-11*cos(psi);
% A(15,12) = 2.63e-10;
% A(13:15,13:15) = -inv_M*D;
% 
A = [Aw zeros(6,9);
    zeros(3,12) Rot_R;
    zeros(3,9) -inv_Tb zeros(3,3);
    zeros(3,6) zeros(3,3) -inv_M*Rot_R' -inv_M*D];

phi = eye(15)+dt*A;
%%

% TAU = dt*E;
P_hat = phi*P*phi' + TAU*Q*TAU';
states_hat = states+dt*F;


%corrector
%kalman gain
K = P_hat*H'/(H*P_hat*H'+R);
% K = zeros(15,3);
P_update = (eye(15)-K*H)*P_hat*(eye(15)-K*H)' + K*R*K';
states_update = states_hat + K*(y-H*states_hat);
error = y - H*states_hat;
end

== matlab function part2_MAIN_2019_for_ayon_because_he_cant_update_his_matlab/ Original/Observer/EKF/MATLAB Function1 ==
  data: states_vector input; eta_hat output; nu_hat output
function [eta_hat, nu_hat] = fcn(states_vector)
%%states [zeta,eta, b, nu] --15x1
%zeta - 6x1, 
%eta - 3x1, 
%b - 3x1, 
%nu - 3x1
eta_hat = states_vector(7:9,1);
nu_hat = states_vector(13:15,1);

end

== matlab function part2_MAIN_2019_for_ayon_because_he_cant_update_his_matlab/ Original/Wind/V_w1/Gust ==
  settings: updateMethod=DISCRETE
  data: time input; u10 input; L input; kappa2 input; gust output
function gust = fcn(time, u10, L, kappa2)

nfreq = 100;
phases = 2*pi * rand(nfreq,1);
gust_tot = 0;
f = zeros(1, nfreq);

for i = 1:nfreq
    f(i) = 0.01 + (i-1)/(nfreq-1) * 0.99;
    f_tilde = L*f(i)/u10;
    S = (4*kappa2*L*u10)/((2+f_tilde^2)^(5/6));
    df = abs(f(2) - f(1));
    gust_part = sqrt(2*S*df)*cos(2*pi*f(i)*time + phases(i));
    gust_tot = gust_tot + gust_part;
end

gust = gust_tot;

== matlab function part2_MAIN_2019_for_ayon_because_he_cant_update_his_matlab/ Original/Wind/V_w1/Mean wind component ==
  data: u10 input; mean_wind output; kappa input; height input
function mean_wind = fcn(u10, kappa, height)
z0 = 10*exp(-2/(5*sqrt(kappa)));
mean_wind = u10 * (5/2) * sqrt(kappa)*log(height/z0);

== matlab function part2_MAIN_2019_for_ayon_because_he_cant_update_his_matlab/ Original/Observer/EKF/Subsystem1/MATLAB Function ==
  data: u input; P1 output; P input; states input; states1 output
function [P1, states1] = fcn(u, P, states)

if u>1
    P1 = eye(15);
    states1 = zeros(15,1);
else
    P1 = P;
    states1 = states;
end

== matlab function part2_MAIN_2019_for_ayon_because_he_cant_update_his_matlab/Simulation 5/Current (North - East)/MATLAB Function ==
  data: u input; y output
function y = fcn(u)
rot = [cos(u) -sin(u) 0;
    sin(u) cos(u) 0;
    0 0 1];

y = rot';

== matlab function part2_MAIN_2019_for_ayon_because_he_cant_update_his_matlab/ Original/Thrust Allocation/MATLAB Function1 ==
  data: tau_d input; Td output; alpha output
function [Td, alpha] = quad_prog_basic_slow(tau_d)
%% x, y, and psi component of tau_d
tau = [tau_d(1); tau_d(2); tau_d(6)]; 

%% Quadratic Programming
% Compute function arguments
% Point to Minimize
u_p = [0 0 0 0 0 0 0 0].'; % [T1 T2x T2y T3 T4x T4y T5x T5y]
u_m = -[0 0 0 0 0 0 0 0].'; % [T1 T2x T2y T3 T4x T4y T5x T5y]
s_p = [0 0 0].'; % [x1 x2 x6]
s_m = -[0 0 0].'; % [x1 x2 x6]
x0 = [u_p; u_m; s_p; s_m]; % auxiliary variables

% persistent x0_l
% 
% % Store previous point
% if isempty(x0_l)
%     x0_l = x0(1:16);
% end

% Objective Function
% Quadratic Objective Term
sWeight = 1e4;
w = [1 1 1 1 0.8 0.8 0.8 0.8]; % Prioritize control over T4 and T5
q = [sWeight sWeight sWeight*10]; % For slackness (Needs Tuning)
H = 2*diag([w w q q]);

% Linear Objective Term
% f = zeros(1, length(x0)); % No linear term in the objective function
f = [];

% Thruster Equality Constraints
% Thruster 1
x1 = 39.3;
y1 = 0;
% Thruster 2
x2 = 35.6;
y2 = 0;
% Thruster 3
x3 = 31.3;
y3 = 0;
% Thruster 4
x4 = -28.5;
y4 = 5;
% Thruster 5
x5 = -28.5;
y5 = -5;

% Redistributed force for each thruster
thr1 = [0 1 x1].';
thr2_x = [1 0 y2].';
thr2_y = [0 1 x2].';
thr3 = [0 1 x3].';
thr4_x = [1 0 y4].';
thr4_y = [0 1 x4].';
thr5_x = [1 0 y5].';
thr5_y = [0 1 x5].';

% B redistributed
B_r = [thr1 thr2_x thr2_y thr3 thr4_x thr4_y thr5_x thr5_y];

Aeq = [B_r -B_r eye(3) -eye(3)];
beq = tau;

% Thruster Saturation Constraints
u_max = [125000, 150000, 150000, 125000, 300000, 300000, 300000, 300000].';
% u_min = [-125000 0 0 -125000 0 0 0 0].';
u_min = -u_max;

% Rate Limitation Constraints
timestep = 0.1;
delta_max = [125000/8*timestep, 150000/8*timestep, 150000/8*timestep, 125000/8*timestep, 300000/10*timestep, 300000/10*timestep, 300000/10*timestep, 300000/10*timestep];
delta_min = -delta_max;

% lim_max = delta_max - x0_l;
% lim_min = delta_min + x0_l;

A = [eye(8) -eye(8) zeros(8,3) zeros(8,3);
     -eye(8) eye(8) zeros(8,3) zeros(8,3)];

% b = [-(max(u_min, lim_min));
%      min(u_max, lim_max)];
b = [-u_min;
    u_max];

lb = [];
ub = [];

options = optimoptions('quadprog', 'Algorithm', 'active-set');

% Compute optimal thruster control
x0_opt = quadprog(H,f,A,b,Aeq,beq,lb,ub,x0, options);

% % Store previous x0_opt
% x0_l = x0_opt(1:16);

% Slack Variable from auxiliary variables
s = x0_opt(17:19) - x0_opt(20:22); % STILL DON'T NOW WHAT TO DO WITH THIS
s_abs = x0_opt(17:19) + x0_opt(20:22); % STILL DON'T NOW WHAT TO DO WITH THIS

% Allocation variables from auxiliary variables
u = x0_opt(1:8) - x0_opt(9:16); 
u_abs = x0_opt(1:8) + x0_opt(9:16); 

%% RESULTS
% Thruster control
Td = [u(1); 
      sqrt(u(2)^2 + u(3)^2); 
      u(4); 
      sqrt(u(5)^2 + u(6)^2);
      sqrt(u(7)^2 + u(8)^2)];

% Thruster angle
alpha2 = atan2(u(3),u(2));
alpha4 = atan2(u(6),u(5));
alpha5 = atan2(u(8),u(7));
alpha = [pi/2; alpha2; pi/2; alpha4; alpha5];
end
% function [Td, alpha] = quad_prog_basic(tau_d)
% %% x, y, and psi component of tau_d
% tau = [tau_d(1); tau_d(2); tau_d(6)]; 
% 
% %% Quadratic Programming
% % Compute function arguments
% % Point to Minimize
% u = [0 0 0 0 0 0 0 0].'; % [T1 T2x T2y T3 T4x T4y T5x T5y]
% s = [0 0 0].'; % [x1 x2 x6]
% x0 = [u; s]; % auxiliary variables
% 
% % persistent x0_l
% % 
% % if isempty(x0_l)
% %     x0_l = x0;
% % end
% 
% % Objective Function
% % Quadratic Objective Term
% sWeight = 1e4;
% w = [1 1 1 1 0.8 0.8 0.8 0.8]; % Prioritize control over T4 and T5
% q = [sWeight sWeight sWeight*10]; % For slackness (Needs Tuning)
% H = 2*diag([w q]);
% 
% % Linear Objective Term
% f = zeros(length(x0),1); % No linear term in the objective function 
% % f = [];
% 
% % Thruster Equality Constraints
% % Thruster 1
% x1 = 39.3;
% y1 = 0;
% % Thruster 2
% x2 = 35.6;
% y2 = 0;
% % Thruster 3
% x3 = 31.3;
% y3 = 0;
% % Thruster 4
% x4 = -28.5;
% y4 = 5;
% % Thruster 5
% x5 = -28.5;
% y5 = -5;
% 
% % Redistributed force for each thruster
% thr1 = [0 1 x1].';
% thr2_x = [1 0 y2].';
% thr2_y = [0 1 x2].';
% thr3 = [0 1 x3].';
% thr4_x = [1 0 y4].';
% thr4_y = [0 1 x4].';
% thr5_x = [1 0 y5].';
% thr5_y = [0 1 x5].';
% 
% % B redistributed
% B_r = [thr1 thr2_x thr2_y thr3 thr4_x thr4_y thr5_x thr5_y];
% 
% Aeq = [B_r, -eye(3)];
% beq = tau;
% 
% % Thruster Saturation Constraints
% u_max = [125000 150000 150000 125000 300000 300000 300000 300000].';
% u_min = -u_max;
% % u_min = [-125000 0 0 -125000 0 0 0 0].';
% 
% A = [-eye(8), zeros(8,3);
%      eye(8), zeros(8,3)];
% 
% b = [-u_min;
%      u_max];
% 
% % coder.extrinsic('quadprog');
% % coder.extrinsic('optimoptions');
% % options = optimoptions('quadprog','Algorithm','interior-point-convex','Display','off','Steptolerance',1e-30,'OptimalityTolerance',1e+3);
% options = optimoptions('quadprog', 'Algorithm', 'active-set');
% % options = optimoptions('quadprog', 'Algorithm', 'interior-point-convex', 'Display', 'iter');
% 
% % Compute optimal thruster control\
% x0_opt = quadprog(H,f,A,b,Aeq,beq,[],[],x0,options);
% 
% % Store previous x0_opt
% % x0_l = x0_opt;
% 
% % Allocation variables from auxiliary variables
% u_f = x0_opt(1:8); 
% 
% %% RESULTS
% % Thruster control
% Td = [u_f(1); 
%       sqrt(u_f(2)^2 + u_f(3)^2); 
%       u_f(4); 
%       sqrt(u_f(5)^2 + u_f(6)^2);
%       sqrt(u_f(7)^2 + u_f(8)^2)];
% 
% % Thruster angle
% alpha2 = atan2(u_f(3),u_f(2));
% alpha4 = atan2(u_f(6),u_f(5));
% alpha5 = atan2(u_f(8),u_f(7));
% alpha = [pi/2; alpha2; pi/2; alpha4; alpha5];
% end
